simulink model "invert"  (R2019a)
settings: Solver=VariableStepAuto  StartTime=0.0  StopTime=10  RelTol=1e-3
settings Model: Creator=dell  LastModifiedBy=dell

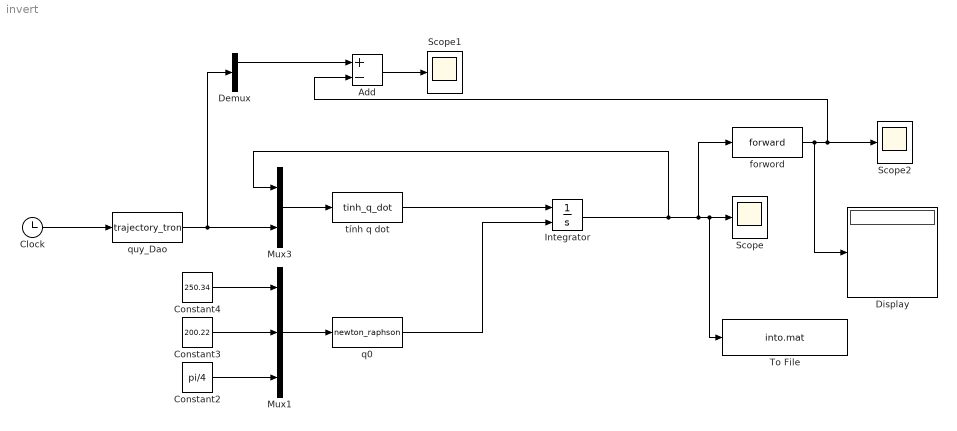
== system invert ==
  Add : Sum  Inputs=+-
  Clock : Clock
  Constant2 : Constant  Value=pi/4
  Constant3 : Constant  Value=200.22
  Constant4 : Constant  Value=250.34
  Demux : Demux  Outputs=2
  Display : Display
      settings: Decimation=3
  Integrator : Integrator  InitialConditionSource=external
  Mux1 : Mux  Inputs=3
  Mux3 : Mux  Inputs=2
  Scope : Scope
  Scope1 : Scope
  Scope2 : Scope
  To File : ToFile  Filename=into.mat
  forword : MATLABFcn  MATLABFcn=forward  OutputDimensions=3
  q0 : MATLABFcn  MATLABFcn=newton_raphson  OutputDimensions=3
  quy_Dao : MATLABFcn  MATLABFcn=trajectory_tron  OutputDimensions=6
  "tính q dot " : MATLABFcn  MATLABFcn=tinh_q_dot  OutputDimensions=3
  wires:
  Mux1/1 -> q0/1
  "tính q dot "/1 -> Integrator/1
  Constant3/1 -> Mux1/2
  Constant4/1 -> Mux1/1
  Constant2/1 -> Mux1/3
  q0/1 -> Integrator/2
  Integrator/1 -> Mux3/1, forword/1, To File/1, Scope/1
  Mux3/1 -> "tính q dot "/1
  quy_Dao/1 -> Demux/1, Mux3/2
  Clock/1 -> quy_Dao/1
  forword/1 -> Display/1, Scope2/1, Add/2
  Demux/1 -> Add/1
  Add/1 -> Scope1/1
